simulink model "GesamtsystemAlt"  (R2018b)
settings: Solver=FixedStepDiscrete  StartTime=0.0  StopTime=1  RelTol=1e-3  EnableMultiTasking=on
libraries: commutil2 x12, c2833xlib x10, c280xlib x8, powerlib_extras x2, simulink x1, c2000lib x1, dspstat3 x1
(part 1 of 3)
settings Model: ExtModeTrigDuration=8  Creator=User  LastModifiedBy=User
settings SolverCC: AutoInsertRateTranBlk=on
settings DataIOCC: LimitDataPoints=on  SaveFormat=Array  SaveOutput=off  SaveTime=off
settings OptimizationCC: DefaultUnderspecifiedDataType=single  ExpressionDepthLimit=2147483647  LifeSpan=1  MaxStackSize=512
settings DebuggingCC: UnderspecifiedInitializationDetection=Classic  MergeDetectMultiDrivingBlocksExec=none  SolverPrmCheckMsg=warning  StateNameClashWarn=warning  SFUnexpectedBacktrackingDiag=warning  SFNoUnconditionalDefaultTransitionDiag=warning  SFExecutionAtInitializationDiag=none
settings HardwareCC: ProdBitPerChar=16  ProdBitPerInt=16  ProdBitPerPointer=32  ProdBitPerSizeT=32  ProdBitPerPtrDiffT=32  ProdLargestAtomicInteger=Integer  ProdLargestAtomicFloat=None  ProdWordSize=16  ProdLongLongMode=on  ProdHWDeviceType=Texas Instruments->C2000  TargetBitPerChar=16  TargetBitPerInt=16  TargetLargestAtomicInteger=Integer  TargetIntDivRoundTo=Zero  TargetEndianess=LittleEndian  TargetWordSize=16  TargetHWDeviceType=Texas Instruments->C2000  ProdEqTarget=off
settings ModelReferenceCC: PropagateSignalLabelsOutOfModel=off
settings SFSimCC: SimCustomSourceCode="#include \"i2c_reset.c\""  SimCustomHeaderCode="#include \"i2c_reset.h\""  SimUseLocalCustomCode=off  MATLABDynamicMemAlloc=off
settings RTWCC: SystemTargetFile=ert.tlc  HardwareBoard=TI Delfino F2833x  TemplateMakefile=ert_default_tmf  RTWUseLocalCustomCode=off  RTWUseSimCustomCode=on  CustomSourceCode="#include \"i2c_reset.c\""  CustomHeaderCode="#include \"i2c_reset.h\""  Toolchain=Texas Instruments Code Composer Studio (C2000)
settings CodeAppCC: IgnoreCustomStorageClasses=off  CustomSymbolStrType=$N$R$M  StateflowObjectComments=on  InternalIdentifier=Classic
settings ERTTargetCC: CodeReplacementLibrary=TI C28x  MultiwordLength=2048  ParMdlRefBuildCompliant=off  SupportContinuousTime=on  CPPClassGenCompliant=off  ConvertIfToSwitch=off  SuppressUnreachableDefaultCases=off
settings ConfigComp: CovMetricSettings=dw  CovHtmlReporting=on  CovSaveCumulativeToWorkspaceVar=on  CovSaveSingleToWorkspaceVar=on  CovExternalEMLEnable=off  PSAutoStubLUT=on

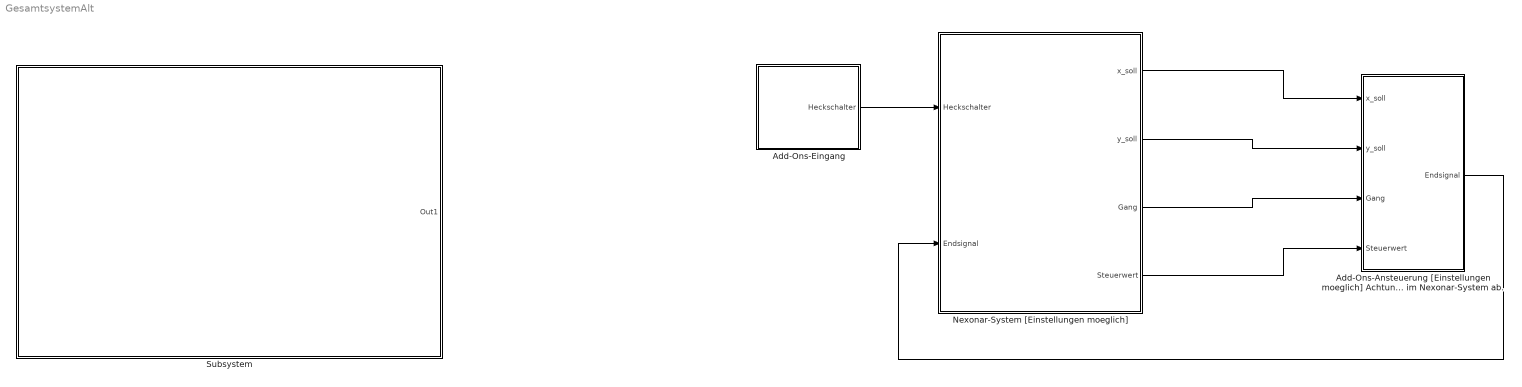
== system GesamtsystemAlt ==
  Add-Ons-Ansteuerung [Einstellungen moeglich] Achtung! Einige Einstellungswerte haengen von den Werten im Nexonar-System ab. : Subsystem
  Add-Ons-Eingang : Subsystem
  Nexonar-System [Einstellungen moeglich] : Subsystem
  Subsystem : Subsystem
  wires:
  Add-Ons-Eingang/1(Heckschalter) -> Nexonar-System [Einstellungen moeglich]/1(Heckschalter)
  Nexonar-System [Einstellungen moeglich]/1(x_soll) -> Add-Ons-Ansteuerung [Einstellungen moeglich] Achtung! Einige Einstellungswerte haengen von den Werten im Nexonar-System ab./1(x_soll)
  Nexonar-System [Einstellungen moeglich]/4(Steuerwert) -> Add-Ons-Ansteuerung [Einstellungen moeglich] Achtung! Einige Einstellungswerte haengen von den Werten im Nexonar-System ab./4(Steuerwert)
  Nexonar-System [Einstellungen moeglich]/3(Gang) -> Add-Ons-Ansteuerung [Einstellungen moeglich] Achtung! Einige Einstellungswerte haengen von den Werten im Nexonar-System ab./3(Gang)
  Nexonar-System [Einstellungen moeglich]/2(y_soll) -> Add-Ons-Ansteuerung [Einstellungen moeglich] Achtung! Einige Einstellungswerte haengen von den Werten im Nexonar-System ab./2(y_soll)
  Add-Ons-Ansteuerung [Einstellungen moeglich] Achtung! Einige Einstellungswerte haengen von den Werten im Nexonar-System ab./1(Endsignal) -> Nexonar-System [Einstellungen moeglich]/2(Endsignal)

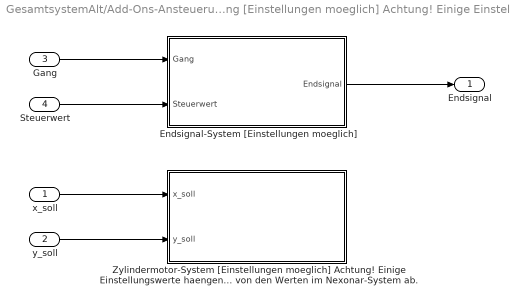
== system GesamtsystemAlt/Add-Ons-Ansteuerung [Einstellungen moeglich] Achtung! Einige Einstellungswerte haengen von den Werten im Nexonar-System ab. ==
  x_soll : Inport
  y_soll : Inport  Port=2
  Gang : Inport  Port=3
  Steuerwert : Inport  Port=4
  Endsignal-System [Einstellungen moeglich] : Subsystem
  Zylindermotor-System [Einstellungen moeglich] Achtung! Einige Einstellungswerte haengen von den Werten im Nexonar-System ab. : Subsystem
  Endsignal : Outport
  wires:
  x_soll/1 -> Zylindermotor-System [Einstellungen moeglich] Achtung! Einige Einstellungswerte haengen von den Werten im Nexonar-System ab./1(x_soll)
  y_soll/1 -> Zylindermotor-System [Einstellungen moeglich] Achtung! Einige Einstellungswerte haengen von den Werten im Nexonar-System ab./2(y_soll)
  Gang/1 -> Endsignal-System [Einstellungen moeglich]/1(Gang)
  Steuerwert/1 -> Endsignal-System [Einstellungen moeglich]/2(Steuerwert)
  Endsignal-System [Einstellungen moeglich]/1(Endsignal) -> Endsignal/1

== system GesamtsystemAlt/Add-Ons-Eingang ==
  Heckschalter-System : Subsystem
  Heckschalter : Outport
  wires:
  Heckschalter-System/1(Heckschalter) -> Heckschalter/1

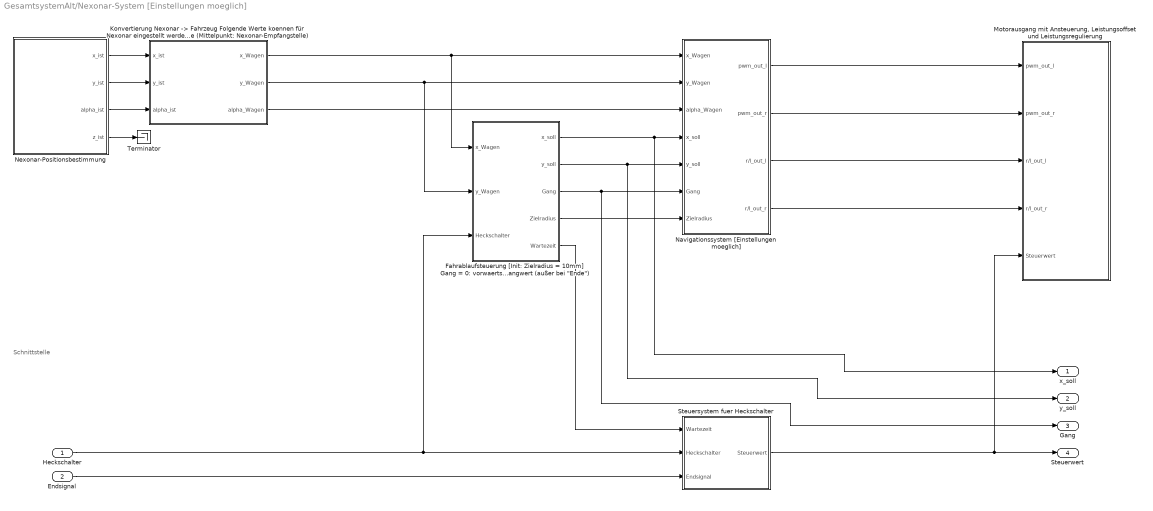
== system GesamtsystemAlt/Nexonar-System [Einstellungen moeglich] ==
  note: Schnittstelle
  Heckschalter : Inport
  Endsignal : Inport  Port=2
  "Fahrablaufsteuerung [Init: Zielradius = 10mm] Gang = 0: vorwaerts Gang = 1: rueckwaerts Folgende Werte fuer den Ablauf sind einstellbar: - Zielkoordinatenwerte - Gangwert (außer bei \"Ende\")" : Stateflow chart  TreatAsAtomicUnit=on
  "Konvertierung Nexonar -> Fahrzeug Folgende Werte koennen für Nexonar eingestellt werden: - r_Versatz_Nexo: Radialer Versatz des Nexonars zur Rotationsachse des Fahrzeugs - phi_Versatz_Nexo: Winkelversatz des Nexonars gegenüber der x-Achse (Mittelpunkt: Rotationspunkt des Fahrzeugs) - psi_Offset_Nexo: Winkelversatz des Nexonars gegenüber der x-Achse (Mittelpunkt: Nexonar-Empfangstelle)" : Stateflow chart  TreatAsAtomicUnit=on
  "Motorausgang mit Ansteuerung, Leistungsoffset und Leistungsregulierung" : Subsystem
  Navigationssystem [Einstellungen moeglich] : Subsystem  TreatAsAtomicUnit=on
  Nexonar-Positionsbestimmung : Subsystem
  Steuersystem fuer Heckschalter : Stateflow chart  TreatAsAtomicUnit=on
  Terminator : Terminator
  x_soll : Outport
  y_soll : Outport  Port=2
  Gang : Outport  Port=3
  Steuerwert : Outport  Port=4
  wires:
  Navigationssystem [Einstellungen moeglich]/3(r/l_out_l) -> "Motorausgang mit Ansteuerung, Leistungsoffset und Leistungsregulierung"/3(r/l_out_l)
  "Konvertierung Nexonar -> Fahrzeug Folgende Werte koennen für Nexonar eingestellt werden: - r_Versatz_Nexo: Radialer Versatz des Nexonars zur Rotationsachse des Fahrzeugs - phi_Versatz_Nexo: Winkelversatz des Nexonars gegenüber der x-Achse (Mittelpunkt: Rotationspunkt des Fahrzeugs) - psi_Offset_Nexo: Winkelversatz des Nexonars gegenüber der x-Achse (Mittelpunkt: Nexonar-Empfangstelle)"/2(y_Wagen) -> "Fahrablaufsteuerung [Init: Zielradius = 10mm] Gang = 0: vorwaerts Gang = 1: rueckwaerts Folgende Werte fuer den Ablauf sind einstellbar: - Zielkoordinatenwerte - Gangwert (außer bei \"Ende\")"/2(y_Wagen), Navigationssystem [Einstellungen moeglich]/2(y_Wagen)
  "Konvertierung Nexonar -> Fahrzeug Folgende Werte koennen für Nexonar eingestellt werden: - r_Versatz_Nexo: Radialer Versatz des Nexonars zur Rotationsachse des Fahrzeugs - phi_Versatz_Nexo: Winkelversatz des Nexonars gegenüber der x-Achse (Mittelpunkt: Rotationspunkt des Fahrzeugs) - psi_Offset_Nexo: Winkelversatz des Nexonars gegenüber der x-Achse (Mittelpunkt: Nexonar-Empfangstelle)"/1(x_Wagen) -> "Fahrablaufsteuerung [Init: Zielradius = 10mm] Gang = 0: vorwaerts Gang = 1: rueckwaerts Folgende Werte fuer den Ablauf sind einstellbar: - Zielkoordinatenwerte - Gangwert (außer bei \"Ende\")"/1(x_Wagen), Navigationssystem [Einstellungen moeglich]/1(x_Wagen)
  Nexonar-Positionsbestimmung/4(z_ist) -> Terminator/1
  Nexonar-Positionsbestimmung/1(x_ist) -> "Konvertierung Nexonar -> Fahrzeug Folgende Werte koennen für Nexonar eingestellt werden: - r_Versatz_Nexo: Radialer Versatz des Nexonars zur Rotationsachse des Fahrzeugs - phi_Versatz_Nexo: Winkelversatz des Nexonars gegenüber der x-Achse (Mittelpunkt: Rotationspunkt des Fahrzeugs) - psi_Offset_Nexo: Winkelversatz des Nexonars gegenüber der x-Achse (Mittelpunkt: Nexonar-Empfangstelle)"/1(x_ist)
  Navigationssystem [Einstellungen moeglich]/4(r/l_out_r) -> "Motorausgang mit Ansteuerung, Leistungsoffset und Leistungsregulierung"/4(r/l_out_r)
  Nexonar-Positionsbestimmung/3(alpha_ist) -> "Konvertierung Nexonar -> Fahrzeug Folgende Werte koennen für Nexonar eingestellt werden: - r_Versatz_Nexo: Radialer Versatz des Nexonars zur Rotationsachse des Fahrzeugs - phi_Versatz_Nexo: Winkelversatz des Nexonars gegenüber der x-Achse (Mittelpunkt: Rotationspunkt des Fahrzeugs) - psi_Offset_Nexo: Winkelversatz des Nexonars gegenüber der x-Achse (Mittelpunkt: Nexonar-Empfangstelle)"/3(alpha_ist)
  "Konvertierung Nexonar -> Fahrzeug Folgende Werte koennen für Nexonar eingestellt werden: - r_Versatz_Nexo: Radialer Versatz des Nexonars zur Rotationsachse des Fahrzeugs - phi_Versatz_Nexo: Winkelversatz des Nexonars gegenüber der x-Achse (Mittelpunkt: Rotationspunkt des Fahrzeugs) - psi_Offset_Nexo: Winkelversatz des Nexonars gegenüber der x-Achse (Mittelpunkt: Nexonar-Empfangstelle)"/3(alpha_Wagen) -> Navigationssystem [Einstellungen moeglich]/3(alpha_Wagen)
  "Fahrablaufsteuerung [Init: Zielradius = 10mm] Gang = 0: vorwaerts Gang = 1: rueckwaerts Folgende Werte fuer den Ablauf sind einstellbar: - Zielkoordinatenwerte - Gangwert (außer bei \"Ende\")"/4(Zielradius) -> Navigationssystem [Einstellungen moeglich]/7(Zielradius)
  Nexonar-Positionsbestimmung/2(y_ist) -> "Konvertierung Nexonar -> Fahrzeug Folgende Werte koennen für Nexonar eingestellt werden: - r_Versatz_Nexo: Radialer Versatz des Nexonars zur Rotationsachse des Fahrzeugs - phi_Versatz_Nexo: Winkelversatz des Nexonars gegenüber der x-Achse (Mittelpunkt: Rotationspunkt des Fahrzeugs) - psi_Offset_Nexo: Winkelversatz des Nexonars gegenüber der x-Achse (Mittelpunkt: Nexonar-Empfangstelle)"/2(y_ist)
  Navigationssystem [Einstellungen moeglich]/1(pwm_out_l) -> "Motorausgang mit Ansteuerung, Leistungsoffset und Leistungsregulierung"/1(pwm_out_l)
  Navigationssystem [Einstellungen moeglich]/2(pwm_out_r) -> "Motorausgang mit Ansteuerung, Leistungsoffset und Leistungsregulierung"/2(pwm_out_r)
  "Fahrablaufsteuerung [Init: Zielradius = 10mm] Gang = 0: vorwaerts Gang = 1: rueckwaerts Folgende Werte fuer den Ablauf sind einstellbar: - Zielkoordinatenwerte - Gangwert (außer bei \"Ende\")"/5(Wartezeit) -> Steuersystem fuer Heckschalter/1(Wartezeit)
  Steuersystem fuer Heckschalter/1(Steuerwert) -> Steuerwert/1, "Motorausgang mit Ansteuerung, Leistungsoffset und Leistungsregulierung"/5(Steuerwert)
  Heckschalter/1 -> Steuersystem fuer Heckschalter/2(Heckschalter), "Fahrablaufsteuerung [Init: Zielradius = 10mm] Gang = 0: vorwaerts Gang = 1: rueckwaerts Folgende Werte fuer den Ablauf sind einstellbar: - Zielkoordinatenwerte - Gangwert (außer bei \"Ende\")"/3(Heckschalter)
  "Fahrablaufsteuerung [Init: Zielradius = 10mm] Gang = 0: vorwaerts Gang = 1: rueckwaerts Folgende Werte fuer den Ablauf sind einstellbar: - Zielkoordinatenwerte - Gangwert (außer bei \"Ende\")"/2(y_soll) -> y_soll/1, Navigationssystem [Einstellungen moeglich]/5(y_soll)
  "Fahrablaufsteuerung [Init: Zielradius = 10mm] Gang = 0: vorwaerts Gang = 1: rueckwaerts Folgende Werte fuer den Ablauf sind einstellbar: - Zielkoordinatenwerte - Gangwert (außer bei \"Ende\")"/3(Gang) -> Gang/1, Navigationssystem [Einstellungen moeglich]/6(Gang)
  "Fahrablaufsteuerung [Init: Zielradius = 10mm] Gang = 0: vorwaerts Gang = 1: rueckwaerts Folgende Werte fuer den Ablauf sind einstellbar: - Zielkoordinatenwerte - Gangwert (außer bei \"Ende\")"/1(x_soll) -> x_soll/1, Navigationssystem [Einstellungen moeglich]/4(x_soll)
  Endsignal/1 -> Steuersystem fuer Heckschalter/3(Endsignal)

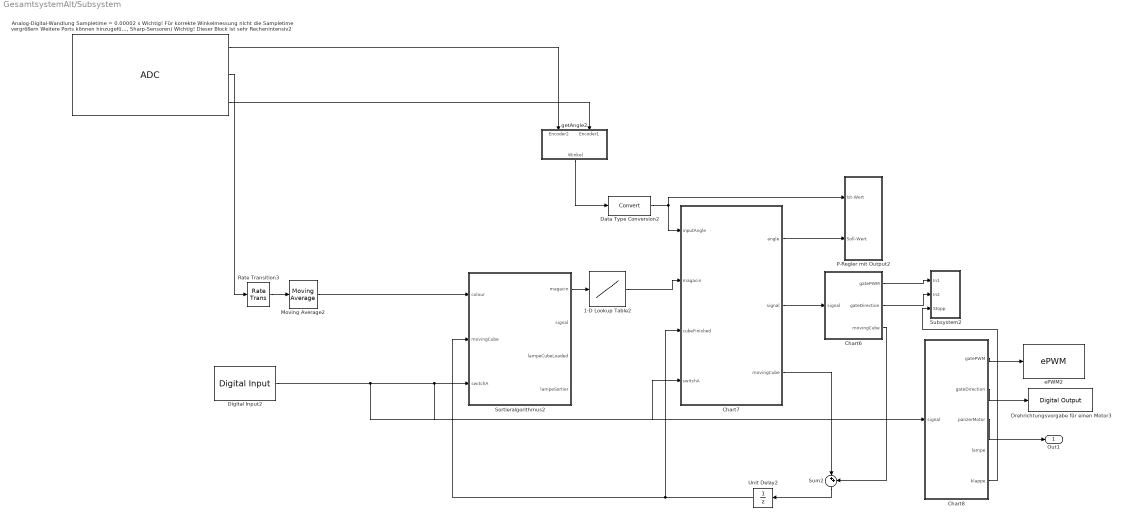
== system GesamtsystemAlt/Subsystem ==
  1-D Lookup Table2 : Lookup_n-D  NumberOfTableDimensions=1  BreakpointsForDimension1=[-1,0,1,2,3,4,5,6]  Table=[-1,-440,-295,-170,-40,85,220,430]  InternalRulePriority=Speed  RndMeth=Simplest  InputSameDT=on
  "Analog-Digital-Wandlung Sampletime = 0.00002 s Wichtig! Für korrekte Winkelmessung nicht die Sampletime vergrößern Weitere Ports können hinzugefügt werden (Farbsensor, Sharp-Sensoren) Wichtig! Dieser Block ist sehr Rechenintensiv2" : c280xlib/ADC  useModule=A  useMode=Sequential  sourceSOC=Software  sourceSOC1=Software  sourceSOC2=ePWMxB  xint2_ADCSOC=31  Ts=0.00002  dType=double  postInterrupt=off  numConversionsSingle=3  numConversionsDouble=1  conv0=ADCINA0  conv1=ADCINA1  conv2=ADCINA2  conv3=ADCINA3  conv4=ADCINA4  conv5=ADCINA5  conv6=ADCINA6  conv7=ADCINA7  conv8=ADCINB0  conv9=ADCINB1  conv10=ADCINB2  conv11=ADCINB3  conv12=ADCINB4  conv13=ADCINB5  conv14=ADCINB6  conv15=ADCINB7  convAB0=ADCINA0 and ADCINB0  convAB1=ADCINA1 and ADCINB1  convAB2=ADCINA2 and ADCINB2  convAB3=ADCINA3 and ADCINB3  convAB4=ADCINA4 and ADCINB4  convAB5=ADCINA5 and ADCINB5  convAB6=ADCINA6 and ADCINB6  convAB7=ADCINA7 and ADCINB7  convA0=ADCINA1  convA1=ADCINA2  convA2=ADCINA0  convA3=ADCINA1  convA4=ADCINA5  convA5=ADCINA5  convA6=ADCINA6  convA7=ADCINA7  convB0=ADCINB0  convB1=ADCINB1  convB2=ADCINB2  convB3=ADCINB3  convB4=ADCINB4  convB5=ADCINB5  convB6=ADCINB6  convB7=ADCINB7  c28xmultiPort=on  endma=off  chdma=1
      settings: SourceProductName=Embedded Coder Support Package for Texas Instruments C2000 Processors  SourceProductBaseCode=TIC2000
  Chart6 : Stateflow chart  TreatAsAtomicUnit=on
  Chart7 : Stateflow chart  TreatAsAtomicUnit=on
  Chart8 : Stateflow chart  TreatAsAtomicUnit=on
  Data Type Conversion2 : DataTypeConversion
  Digital Input2 : c2833xlib/Digital Input  GPIO_Number=GPIO24~GPIO31  GPIO_Bit0=on  GPIO_Bit1=off  GPIO_Bit2=off  GPIO_Bit3=off  GPIO_Bit4=off  GPIO_Bit5=off  GPIO_Bit6=off  GPIO_Bit7=off  sampleTime=0.1  dataType=auto  GPIO_Bit0_Qualification=Sync to SYSCLKOUT  GPIO_Bit1_Qualification=Sync to SYSCLKOUT  GPIO_Bit2_Qualification=Sync to SYSCLKOUT  GPIO_Bit3_Qualification=Sync to SYSCLKOUT  GPIO_Bit4_Qualification=Sync to SYSCLKOUT  GPIO_Bit5_Qualification=Sync to SYSCLKOUT  GPIO_Bit6_Qualification=Sync to SYSCLKOUT  GPIO_Bit7_Qualification=Sync to SYSCLKOUT  Qualification_Period=-1
      settings: SourceProductName=Embedded Coder Support Package for Texas Instruments C2000 Processors  SourceProductBaseCode=TIC2000
  Drehrichtungsvorgabe für einen Motor3 : c2833xlib/Digital Output  GPIO_Number=GPIO8~GPIO15  GPIO_Bit0=off  GPIO_BIT0_Toggle=off  GPIO_Bit1=off  GPIO_BIT1_Toggle=off  GPIO_Bit2=off  GPIO_BIT2_Toggle=off  GPIO_Bit3=off  GPIO_BIT3_Toggle=off  GPIO_Bit4=off  GPIO_BIT4_Toggle=off  GPIO_Bit5=off  GPIO_BIT5_Toggle=off  GPIO_Bit6=off  GPIO_BIT6_Toggle=off  GPIO_Bit7=on  GPIO_BIT7_Toggle=off
      settings: SourceProductName=Embedded Coder Support Package for Texas Instruments C2000 Processors  SourceProductBaseCode=TIC2000
  Moving Average2 : dspstat3/Moving Average  Method=Exponential weighting  ForgettingFactorPort=off  SpecifyWindowLength=on  WindowLength=4  ForgettingFactor=0.3  SimulateUsing=Code generation
  P-Regler mit Output2 : Subsystem
  Rate Transition3 : RateTransition  OutPortSampleTime=0.01
  Sortieralgorithmus2 : Stateflow chart  TreatAsAtomicUnit=on
  Subsystem2 : Subsystem
  Sum2 : Sum  Inputs=|++
  Unit Delay2 : UnitDelay  SampleTime=-1
  ePWM2 : c280xlib/ePWM  checkMode=off  useModule=ePWM5  periodUnits=Clock cycles  timerSource=Specify via dialog  timerPeriod_clk=64000  timerPeriod_sec=0.0001  tbshadow=Counter equals to zero  countingMode=Up  phaseActiveEnable=Disable  phaseDirection=Count down after sync  phaseActive=0  synchronizationEnable=off  synchronizationOption=Disable  clockPrescale=1  HSclockPrescale=1  ePWMxAStatus=off  CMPAUnits=Clock cycles  CMPASource=Specify via dialog  CMPAValue_per=50  CMPAValue_clk=32000  enCMPAshadow=Counter equals to zero  ePWMxAactionLogic1=Do nothing  ePWMxAactionLogic2=Clear  ePWMxAactionLogic3=Set  ePWMxAactionLogic4=Do nothing  ePWMxAactionLogic5=Do nothing  ePWMxAactionLogic6=Do nothing  ePWMxALoadMode=Load on counter equals to zero (CTR=Zero)  ePWMxACSFenable=off  ePWMxACSFvalue=Forcing disable  ePWMxASFreload=Zero  enHRPWM=off  HRPWM_LoadMode=Counter equals to zero (CTR=ZERO)  HRPWM_CTLMode=Phase control mode  HRPWM_EDGMode=Both edge  enSFO=on  ePWMxBStatus=on  CMPBUnits=Percentages  CMPBSource=Input port  CMPBValue_per=50  CMPBValue_clk=32000  enCMPBshadow=Counter equals to zero  ePWMxBactionLogic1=Do nothing  ePWMxBactionLogic2=Set  ePWMxBactionLogic3=Do nothing  ePWMxBactionLogic4=Do nothing  ePWMxBactionLogic5=Clear  ePWMxBactionLogic6=Do nothing  ePWMxBLoadMode=Load on counter equals to zero (CTR=Zero)  ePWMxBCSFenable=off  ePWMxBCSFvalue=Forcing disable  ePWMxBSFreload=Zero  enableDBePWMxA=off  enableDBePWMxB=off  DBpolarity=Active high (AH)  DBedgeDelay=Positive  DBSource_ePWMxA=ePWMxA  DBSource_ePWMxB=ePWMxA  DBperiodSource=Specify via dialog  REDperiod=0  FEDperiod=0  adcstartModuleA=off  adcrequestEventA=First event  adcstartEventA=Counter equals to zero (CTR=Zero)  adcstartModuleB=off  adcrequestEventB=First event  adcstartEventB=Counter equals to zero (CTR=Zero)  intEn=off  intPrd=First event  intSel=Counter equals to zero (CTR=Zero)  chopperEnable=off  chopperFrequency=1  chopperFirstwidth=1  chopperDuty=12.5%  tripZonesource=Specify via dialog  tzselOSHT1=off  tzselOSHT2=off  tzselOSHT3=off  tzselOSHT4=off  tzselOSHT5=off  tzselOSHT6=off  tzselCBC1=off  tzselCBC2=off  tzselCBC3=off  tzselCBC4=off  tzselCBC5=off  tzselCBC6=off  enTzOstIntr=off  enTzCbcIntr=off  ePWMxAforced=No action  ePWMxBforced=No action  timerPeriod=-1  ePWMxAValue=0  ePWMxBValue=0  tripZoneoption=One-shot trip (OSHT)
      settings: SourceProductName=Embedded Coder Support Package for Texas Instruments C2000 Processors  SourceProductBaseCode=TIC2000
  getAngle2 : Subsystem
  Out1 : Outport
  wires:
  Moving Average2/1 -> Sortieralgorithmus2/1(colour)
  Chart8/1(gatePWM) -> ePWM2/1
  getAngle2/1(Winkel) -> Data Type Conversion2/1
  Chart6/3(movingCube) -> Sum2/2
  "Analog-Digital-Wandlung Sampletime = 0.00002 s Wichtig! Für korrekte Winkelmessung nicht die Sampletime vergrößern Weitere Ports können hinzugefügt werden (Farbsensor, Sharp-Sensoren) Wichtig! Dieser Block ist sehr Rechenintensiv2"/2 -> Rate Transition3/1
  Digital Input2/1 -> Chart7/4(switchA), Chart8/1(signal), Sortieralgorithmus2/3(switchA)
  Chart6/1(gatePWM) -> Subsystem2/1(In1)
  Chart8/2(gateDirection) -> Drehrichtungsvorgabe für einen Motor3/1
  Chart7/1(angle) -> P-Regler mit Output2/2(Soll-Wert)
  Rate Transition3/1 -> Moving Average2/1
  Unit Delay2/1 -> Chart7/3(cubeFinished), Sortieralgorithmus2/2(movingCube)
  Chart6/2(gateDirection) -> Subsystem2/2(In2)
  Data Type Conversion2/1 -> Chart7/1(inputAngle), P-Regler mit Output2/1(Ist-Wert)
  Sortieralgorithmus2/1(magacin) -> 1-D Lookup Table2/1
  Chart7/2(signal) -> Chart6/1(signal)
  1-D Lookup Table2/1 -> Chart7/2(magacin)
  "Analog-Digital-Wandlung Sampletime = 0.00002 s Wichtig! Für korrekte Winkelmessung nicht die Sampletime vergrößern Weitere Ports können hinzugefügt werden (Farbsensor, Sharp-Sensoren) Wichtig! Dieser Block ist sehr Rechenintensiv2"/1 -> getAngle2/1(Encoder2)
  Sum2/1 -> Unit Delay2/1
  Chart7/3(movingCube) -> Sum2/1
  "Analog-Digital-Wandlung Sampletime = 0.00002 s Wichtig! Für korrekte Winkelmessung nicht die Sampletime vergrößern Weitere Ports können hinzugefügt werden (Farbsensor, Sharp-Sensoren) Wichtig! Dieser Block ist sehr Rechenintensiv2"/3 -> getAngle2/2(Encoder1)
  Chart8/3(panzerMotor) -> Out1/1
  Chart8/5(klappe) -> Subsystem2/3("Stopp ")

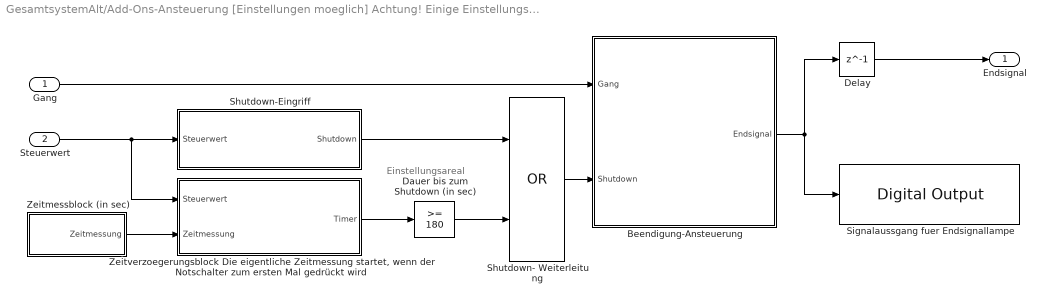
== system GesamtsystemAlt/Add-Ons-Ansteuerung [Einstellungen moeglich] Achtung! Einige Einstellungswerte haengen von den Werten im Nexonar-System ab./Endsignal-System [Einstellungen moeglich] ==
  note: Einstellungsareal
  Gang : Inport
  Steuerwert : Inport  Port=2
  Beendigung-Ansteuerung : Stateflow chart  TreatAsAtomicUnit=on
  Dauer bis zum Shutdown (in sec) : simulink/Logic and Bit Operations/Compare To Constant  relop=>=  const=180  OutDataTypeStr=boolean
  Delay : Delay  DelayLength=1  InitialCondition=0
  Shutdown- Weiterleitung : Logic  Operator=OR  AllPortsSameDT=off  OutDataTypeStr=boolean
  Shutdown-Eingriff : Stateflow chart  TreatAsAtomicUnit=on
  Signalaussgang fuer Endsignallampe : c2833xlib/Digital Output  GPIO_Number=GPIO56~GPIO63  GPIO_Bit0=off  GPIO_BIT0_Toggle=off  GPIO_Bit1=off  GPIO_BIT1_Toggle=off  GPIO_Bit2=on  GPIO_BIT2_Toggle=off  GPIO_Bit3=off  GPIO_BIT3_Toggle=off  GPIO_Bit4=off  GPIO_BIT4_Toggle=off  GPIO_Bit5=off  GPIO_BIT5_Toggle=off  GPIO_Bit6=off  GPIO_BIT6_Toggle=off  GPIO_Bit7=off  GPIO_BIT7_Toggle=off
      settings: SourceProductName=Embedded Coder Support Package for Texas Instruments C2000 Processors  SourceProductBaseCode=TIC2000
  Zeitmessblock (in sec) : Subsystem
  "Zeitverzoegerungsblock Die eigentliche Zeitmessung startet, wenn der Notschalter zum ersten Mal gedrückt wird" : Stateflow chart  TreatAsAtomicUnit=on
  Endsignal : Outport
  wires:
  Gang/1 -> Beendigung-Ansteuerung/1(Gang)
  Beendigung-Ansteuerung/1(Endsignal) -> Signalaussgang fuer Endsignallampe/1, Delay/1
  "Zeitverzoegerungsblock Die eigentliche Zeitmessung startet, wenn der Notschalter zum ersten Mal gedrückt wird"/1(Timer) -> Dauer bis zum Shutdown (in sec)/1
  Steuerwert/1 -> "Zeitverzoegerungsblock Die eigentliche Zeitmessung startet, wenn der Notschalter zum ersten Mal gedrückt wird"/1(Steuerwert), Shutdown-Eingriff/1(Steuerwert)
  Zeitmessblock (in sec)/1(Zeitmessung) -> "Zeitverzoegerungsblock Die eigentliche Zeitmessung startet, wenn der Notschalter zum ersten Mal gedrückt wird"/2(Zeitmessung)
  Delay/1 -> Endsignal/1
  Shutdown- Weiterleitung/1 -> Beendigung-Ansteuerung/2(Shutdown)
  Dauer bis zum Shutdown (in sec)/1 -> Shutdown- Weiterleitung/2
  Shutdown-Eingriff/1(Shutdown) -> Shutdown- Weiterleitung/1

== system GesamtsystemAlt/Add-Ons-Ansteuerung [Einstellungen moeglich] Achtung! Einige Einstellungswerte haengen von den Werten im Nexonar-System ab./Zylindermotor-System [Einstellungen moeglich] Achtung! Einige Einstellungswerte haengen von den Werten im Nexonar-System ab. ==
  x_soll : Inport
  y_soll : Inport  Port=2
  Drehrichtungsvorgabe für Zylindermotor : c2833xlib/Digital Output  GPIO_Number=GPIO16~GPIO23  GPIO_Bit0=off  GPIO_BIT0_Toggle=off  GPIO_Bit1=on  GPIO_BIT1_Toggle=off  GPIO_Bit2=off  GPIO_BIT2_Toggle=off  GPIO_Bit3=off  GPIO_BIT3_Toggle=off  GPIO_Bit4=off  GPIO_BIT4_Toggle=off  GPIO_Bit5=off  GPIO_BIT5_Toggle=off  GPIO_Bit6=off  GPIO_BIT6_Toggle=off  GPIO_Bit7=off  GPIO_BIT7_Toggle=off
      settings: SourceProductName=Embedded Coder Support Package for Texas Instruments C2000 Processors  SourceProductBaseCode=TIC2000
  PWM Vorgabe für Zylindermotor : c280xlib/ePWM  checkMode=off  useModule=ePWM3  periodUnits=Clock cycles  timerSource=Specify via dialog  timerPeriod_clk=64000  timerPeriod_sec=0.0001  tbshadow=Counter equals to zero  countingMode=Up  phaseActiveEnable=Disable  phaseDirection=Count down after sync  phaseActive=0  synchronizationEnable=off  synchronizationOption=Disable  clockPrescale=1  HSclockPrescale=1  ePWMxAStatus=off  CMPAUnits=Clock cycles  CMPASource=Specify via dialog  CMPAValue_per=50  CMPAValue_clk=32000  enCMPAshadow=Counter equals to zero  ePWMxAactionLogic1=Do nothing  ePWMxAactionLogic2=Clear  ePWMxAactionLogic3=Set  ePWMxAactionLogic4=Do nothing  ePWMxAactionLogic5=Do nothing  ePWMxAactionLogic6=Do nothing  ePWMxALoadMode=Load on counter equals to zero (CTR=Zero)  ePWMxACSFenable=off  ePWMxACSFvalue=Forcing disable  ePWMxASFreload=Zero  enHRPWM=off  HRPWM_LoadMode=Counter equals to zero (CTR=ZERO)  HRPWM_CTLMode=Phase control mode  HRPWM_EDGMode=Both edge  enSFO=on  ePWMxBStatus=on  CMPBUnits=Percentages  CMPBSource=Input port  CMPBValue_per=0  CMPBValue_clk=32000  enCMPBshadow=Counter equals to zero  ePWMxBactionLogic1=Do nothing  ePWMxBactionLogic2=Set  ePWMxBactionLogic3=Do nothing  ePWMxBactionLogic4=Do nothing  ePWMxBactionLogic5=Clear  ePWMxBactionLogic6=Do nothing  ePWMxBLoadMode=Load on counter equals to zero (CTR=Zero)  ePWMxBCSFenable=off  ePWMxBCSFvalue=Forcing disable  ePWMxBSFreload=Zero  enableDBePWMxA=off  enableDBePWMxB=off  DBpolarity=Active high (AH)  DBedgeDelay=Positive  DBSource_ePWMxA=ePWMxA  DBSource_ePWMxB=ePWMxA  DBperiodSource=Specify via dialog  REDperiod=0  FEDperiod=0  adcstartModuleA=off  adcrequestEventA=First event  adcstartEventA=Counter equals to zero (CTR=Zero)  adcstartModuleB=off  adcrequestEventB=First event  adcstartEventB=Counter equals to zero (CTR=Zero)  intEn=off  intPrd=First event  intSel=Counter equals to zero (CTR=Zero)  chopperEnable=off  chopperFrequency=1  chopperFirstwidth=1  chopperDuty=12.5%  tripZonesource=Specify via dialog  tzselOSHT1=off  tzselOSHT2=off  tzselOSHT3=off  tzselOSHT4=off  tzselOSHT5=off  tzselOSHT6=off  tzselCBC1=off  tzselCBC2=off  tzselCBC3=off  tzselCBC4=off  tzselCBC5=off  tzselCBC6=off  enTzOstIntr=off  enTzCbcIntr=off  ePWMxAforced=No action  ePWMxBforced=No action  timerPeriod=-1  ePWMxAValue=0  ePWMxBValue=0  tripZoneoption=One-shot trip (OSHT)
      settings: SourceProductName=Embedded Coder Support Package for Texas Instruments C2000 Processors  SourceProductBaseCode=TIC2000
  "Zylindermotor-Ansteuerung Folgende Werte sind einstellbar: - Drehstaerke (in %) (-> ZM_pwm_out in \"Ausfuerung\") - Drehrichtung (rechts = 0, links = 1) (-> ZM_r_l_out in \"Init_und_Warten\") - Drehdauer (-> zwischen \"Ausfuehrung\" und \"Beendet\") - Ausfuehrungspunkt (in mm) [durch Wechsel der Soll-Position] (-> zwischen \"Init_und_Start\" und \"Ausfuehrung) Wichtig! Der Ausfuerungspunkt haengt von den EXAKTEN Soll-Werten aus der Fahrablaufsteuerung im Nexonar-System ab." : Stateflow chart  TreatAsAtomicUnit=on
  wires:
  "Zylindermotor-Ansteuerung Folgende Werte sind einstellbar: - Drehstaerke (in %) (-> ZM_pwm_out in \"Ausfuerung\") - Drehrichtung (rechts = 0, links = 1) (-> ZM_r_l_out in \"Init_und_Warten\") - Drehdauer (-> zwischen \"Ausfuehrung\" und \"Beendet\") - Ausfuehrungspunkt (in mm) [durch Wechsel der Soll-Position] (-> zwischen \"Init_und_Start\" und \"Ausfuehrung) Wichtig! Der Ausfuerungspunkt haengt von den EXAKTEN Soll-Werten aus der Fahrablaufsteuerung im Nexonar-System ab."/1(ZM_pwm_out) -> PWM Vorgabe für Zylindermotor/1
  "Zylindermotor-Ansteuerung Folgende Werte sind einstellbar: - Drehstaerke (in %) (-> ZM_pwm_out in \"Ausfuerung\") - Drehrichtung (rechts = 0, links = 1) (-> ZM_r_l_out in \"Init_und_Warten\") - Drehdauer (-> zwischen \"Ausfuehrung\" und \"Beendet\") - Ausfuehrungspunkt (in mm) [durch Wechsel der Soll-Position] (-> zwischen \"Init_und_Start\" und \"Ausfuehrung) Wichtig! Der Ausfuerungspunkt haengt von den EXAKTEN Soll-Werten aus der Fahrablaufsteuerung im Nexonar-System ab."/2(ZM_r_l_out) -> Drehrichtungsvorgabe für Zylindermotor/1
  y_soll/1 -> "Zylindermotor-Ansteuerung Folgende Werte sind einstellbar: - Drehstaerke (in %) (-> ZM_pwm_out in \"Ausfuerung\") - Drehrichtung (rechts = 0, links = 1) (-> ZM_r_l_out in \"Init_und_Warten\") - Drehdauer (-> zwischen \"Ausfuehrung\" und \"Beendet\") - Ausfuehrungspunkt (in mm) [durch Wechsel der Soll-Position] (-> zwischen \"Init_und_Start\" und \"Ausfuehrung) Wichtig! Der Ausfuerungspunkt haengt von den EXAKTEN Soll-Werten aus der Fahrablaufsteuerung im Nexonar-System ab."/2(y_soll)
  x_soll/1 -> "Zylindermotor-Ansteuerung Folgende Werte sind einstellbar: - Drehstaerke (in %) (-> ZM_pwm_out in \"Ausfuerung\") - Drehrichtung (rechts = 0, links = 1) (-> ZM_r_l_out in \"Init_und_Warten\") - Drehdauer (-> zwischen \"Ausfuehrung\" und \"Beendet\") - Ausfuehrungspunkt (in mm) [durch Wechsel der Soll-Position] (-> zwischen \"Init_und_Start\" und \"Ausfuehrung) Wichtig! Der Ausfuerungspunkt haengt von den EXAKTEN Soll-Werten aus der Fahrablaufsteuerung im Nexonar-System ab."/1(x_soll)

== system GesamtsystemAlt/Add-Ons-Eingang/Heckschalter-System ==
  Signaleingang fuer Heckschalter : c2833xlib/Digital Input  GPIO_Number=GPIO24~GPIO31  GPIO_Bit0=on  GPIO_Bit1=off  GPIO_Bit2=off  GPIO_Bit3=off  GPIO_Bit4=off  GPIO_Bit5=off  GPIO_Bit6=off  GPIO_Bit7=off  sampleTime=0.01  dataType=boolean  GPIO_Bit0_Qualification=Sync to SYSCLKOUT  GPIO_Bit1_Qualification=Sync to SYSCLKOUT  GPIO_Bit2_Qualification=Sync to SYSCLKOUT  GPIO_Bit3_Qualification=Sync to SYSCLKOUT  GPIO_Bit4_Qualification=Sync to SYSCLKOUT  GPIO_Bit5_Qualification=Sync to SYSCLKOUT  GPIO_Bit6_Qualification=Sync to SYSCLKOUT  GPIO_Bit7_Qualification=Sync to SYSCLKOUT  Qualification_Period=-1
      settings: SourceProductName=Embedded Coder Support Package for Texas Instruments C2000 Processors  SourceProductBaseCode=TIC2000
  Heckschalter : Outport
  wires:
  Signaleingang fuer Heckschalter/1 -> Heckschalter/1

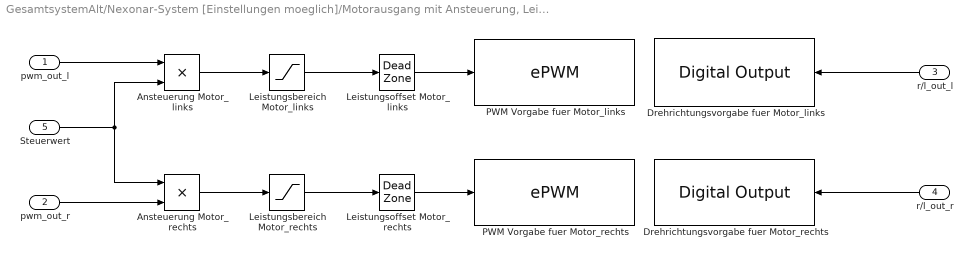
== system GesamtsystemAlt/Nexonar-System [Einstellungen moeglich]/Motorausgang mit Ansteuerung, Leistungsoffset und Leistungsregulierung ==
  pwm_out_l : Inport
  pwm_out_r : Inport  Port=2
  r/l_out_l : Inport  Port=3
  r/l_out_r : Inport  Port=4
  Steuerwert : Inport  Port=5
  Ansteuerung Motor_links : Product
  Ansteuerung Motor_rechts : Product
  Drehrichtungsvorgabe fuer Motor_links : c2833xlib/Digital Output  GPIO_Number=GPIO16~GPIO23  GPIO_Bit0=off  GPIO_BIT0_Toggle=off  GPIO_Bit1=off  GPIO_BIT1_Toggle=off  GPIO_Bit2=off  GPIO_BIT2_Toggle=off  GPIO_Bit3=off  GPIO_BIT3_Toggle=off  GPIO_Bit4=on  GPIO_BIT4_Toggle=off  GPIO_Bit5=off  GPIO_BIT5_Toggle=off  GPIO_Bit6=off  GPIO_BIT6_Toggle=off  GPIO_Bit7=off  GPIO_BIT7_Toggle=off
      settings: SourceProductName=Embedded Coder Support Package for Texas Instruments C2000 Processors  SourceProductBaseCode=TIC2000
  Drehrichtungsvorgabe fuer Motor_rechts : c2833xlib/Digital Output  GPIO_Number=GPIO16~GPIO23  GPIO_Bit0=off  GPIO_BIT0_Toggle=off  GPIO_Bit1=off  GPIO_BIT1_Toggle=off  GPIO_Bit2=off  GPIO_BIT2_Toggle=off  GPIO_Bit3=off  GPIO_BIT3_Toggle=off  GPIO_Bit4=off  GPIO_BIT4_Toggle=off  GPIO_Bit5=on  GPIO_BIT5_Toggle=off  GPIO_Bit6=off  GPIO_BIT6_Toggle=off  GPIO_Bit7=off  GPIO_BIT7_Toggle=off
      settings: SourceProductName=Embedded Coder Support Package for Texas Instruments C2000 Processors  SourceProductBaseCode=TIC2000
  Leistungsbereich Motor_links : Saturate  UpperLimit=80  LowerLimit=0
  Leistungsbereich Motor_rechts : Saturate  UpperLimit=80  LowerLimit=0
  Leistungsoffset Motor_links : DeadZone  LowerValue=0  UpperValue=0  SaturateOnIntegerOverflow=on
  Leistungsoffset Motor_rechts : DeadZone  LowerValue=0  UpperValue=3  SaturateOnIntegerOverflow=on
  "PWM Vorgabe fuer Motor_links " : c280xlib/ePWM  checkMode=off  useModule=ePWM1  periodUnits=Clock cycles  timerSource=Specify via dialog  timerPeriod_clk=64000  timerPeriod_sec=0.0001  tbshadow=Counter equals to zero  countingMode=Up  phaseActiveEnable=Disable  phaseDirection=Count down after sync  phaseActive=0  synchronizationEnable=off  synchronizationOption=Disable  clockPrescale=1  HSclockPrescale=1  ePWMxAStatus=off  CMPAUnits=Clock cycles  CMPASource=Specify via dialog  CMPAValue_per=50  CMPAValue_clk=32000  enCMPAshadow=Counter equals to zero  ePWMxAactionLogic1=Do nothing  ePWMxAactionLogic2=Clear  ePWMxAactionLogic3=Set  ePWMxAactionLogic4=Do nothing  ePWMxAactionLogic5=Do nothing  ePWMxAactionLogic6=Do nothing  ePWMxALoadMode=Load on counter equals to zero (CTR=Zero)  ePWMxACSFenable=off  ePWMxACSFvalue=Forcing disable  ePWMxASFreload=Zero  enHRPWM=off  HRPWM_LoadMode=Counter equals to zero (CTR=ZERO)  HRPWM_CTLMode=Phase control mode  HRPWM_EDGMode=Both edge  enSFO=on  ePWMxBStatus=on  CMPBUnits=Percentages  CMPBSource=Input port  CMPBValue_per=0  CMPBValue_clk=32000  enCMPBshadow=Counter equals to zero  ePWMxBactionLogic1=Do nothing  ePWMxBactionLogic2=Set  ePWMxBactionLogic3=Do nothing  ePWMxBactionLogic4=Do nothing  ePWMxBactionLogic5=Clear  ePWMxBactionLogic6=Do nothing  ePWMxBLoadMode=Load on counter equals to zero (CTR=Zero)  ePWMxBCSFenable=off  ePWMxBCSFvalue=Forcing disable  ePWMxBSFreload=Zero  enableDBePWMxA=off  enableDBePWMxB=off  DBpolarity=Active high (AH)  DBedgeDelay=Positive  DBSource_ePWMxA=ePWMxA  DBSource_ePWMxB=ePWMxA  DBperiodSource=Specify via dialog  REDperiod=0  FEDperiod=0  adcstartModuleA=off  adcrequestEventA=First event  adcstartEventA=Counter equals to zero (CTR=Zero)  adcstartModuleB=off  adcrequestEventB=First event  adcstartEventB=Counter equals to zero (CTR=Zero)  intEn=off  intPrd=First event  intSel=Counter equals to zero (CTR=Zero)  chopperEnable=off  chopperFrequency=1  chopperFirstwidth=1  chopperDuty=12.5%  tripZonesource=Specify via dialog  tzselOSHT1=off  tzselOSHT2=off  tzselOSHT3=off  tzselOSHT4=off  tzselOSHT5=off  tzselOSHT6=off  tzselCBC1=off  tzselCBC2=off  tzselCBC3=off  tzselCBC4=off  tzselCBC5=off  tzselCBC6=off  enTzOstIntr=off  enTzCbcIntr=off  ePWMxAforced=No action  ePWMxBforced=No action  timerPeriod=-1  ePWMxAValue=0  ePWMxBValue=0  tripZoneoption=One-shot trip (OSHT)
      settings: SourceProductName=Embedded Coder Support Package for Texas Instruments C2000 Processors  SourceProductBaseCode=TIC2000
  PWM Vorgabe fuer Motor_rechts : c280xlib/ePWM  checkMode=off  useModule=ePWM2  periodUnits=Clock cycles  timerSource=Specify via dialog  timerPeriod_clk=64000  timerPeriod_sec=0.0001  tbshadow=Counter equals to zero  countingMode=Up  phaseActiveEnable=Disable  phaseDirection=Count down after sync  phaseActive=0  synchronizationEnable=off  synchronizationOption=Disable  clockPrescale=1  HSclockPrescale=1  ePWMxAStatus=off  CMPAUnits=Clock cycles  CMPASource=Specify via dialog  CMPAValue_per=50  CMPAValue_clk=32000  enCMPAshadow=Counter equals to zero  ePWMxAactionLogic1=Do nothing  ePWMxAactionLogic2=Clear  ePWMxAactionLogic3=Set  ePWMxAactionLogic4=Do nothing  ePWMxAactionLogic5=Do nothing  ePWMxAactionLogic6=Do nothing  ePWMxALoadMode=Load on counter equals to zero (CTR=Zero)  ePWMxACSFenable=off  ePWMxACSFvalue=Forcing disable  ePWMxASFreload=Zero  enHRPWM=off  HRPWM_LoadMode=Counter equals to zero (CTR=ZERO)  HRPWM_CTLMode=Phase control mode  HRPWM_EDGMode=Both edge  enSFO=on  ePWMxBStatus=on  CMPBUnits=Percentages  CMPBSource=Input port  CMPBValue_per=0  CMPBValue_clk=32000  enCMPBshadow=Counter equals to zero  ePWMxBactionLogic1=Do nothing  ePWMxBactionLogic2=Set  ePWMxBactionLogic3=Do nothing  ePWMxBactionLogic4=Do nothing  ePWMxBactionLogic5=Clear  ePWMxBactionLogic6=Do nothing  ePWMxBLoadMode=Load on counter equals to zero (CTR=Zero)  ePWMxBCSFenable=off  ePWMxBCSFvalue=Forcing disable  ePWMxBSFreload=Zero  enableDBePWMxA=off  enableDBePWMxB=off  DBpolarity=Active high (AH)  DBedgeDelay=Positive  DBSource_ePWMxA=ePWMxA  DBSource_ePWMxB=ePWMxA  DBperiodSource=Specify via dialog  REDperiod=0  FEDperiod=0  adcstartModuleA=off  adcrequestEventA=First event  adcstartEventA=Counter equals to zero (CTR=Zero)  adcstartModuleB=off  adcrequestEventB=First event  adcstartEventB=Counter equals to zero (CTR=Zero)  intEn=off  intPrd=First event  intSel=Counter equals to zero (CTR=Zero)  chopperEnable=off  chopperFrequency=1  chopperFirstwidth=1  chopperDuty=12.5%  tripZonesource=Specify via dialog  tzselOSHT1=off  tzselOSHT2=off  tzselOSHT3=off  tzselOSHT4=off  tzselOSHT5=off  tzselOSHT6=off  tzselCBC1=off  tzselCBC2=off  tzselCBC3=off  tzselCBC4=off  tzselCBC5=off  tzselCBC6=off  enTzOstIntr=off  enTzCbcIntr=off  ePWMxAforced=No action  ePWMxBforced=No action  timerPeriod=-1  ePWMxAValue=0  ePWMxBValue=0  tripZoneoption=One-shot trip (OSHT)
      settings: SourceProductName=Embedded Coder Support Package for Texas Instruments C2000 Processors  SourceProductBaseCode=TIC2000
  wires:
  pwm_out_l/1 -> Ansteuerung Motor_links/1
  pwm_out_r/1 -> Ansteuerung Motor_rechts/2
  r/l_out_l/1 -> Drehrichtungsvorgabe fuer Motor_links/1
  r/l_out_r/1 -> Drehrichtungsvorgabe fuer Motor_rechts/1
  Leistungsoffset Motor_links/1 -> "PWM Vorgabe fuer Motor_links "/1
  Leistungsoffset Motor_rechts/1 -> PWM Vorgabe fuer Motor_rechts/1
  Steuerwert/1 -> Ansteuerung Motor_rechts/1, Ansteuerung Motor_links/2
  Ansteuerung Motor_rechts/1 -> Leistungsbereich Motor_rechts/1
  Leistungsbereich Motor_rechts/1 -> Leistungsoffset Motor_rechts/1
  Ansteuerung Motor_links/1 -> Leistungsbereich Motor_links/1
  Leistungsbereich Motor_links/1 -> Leistungsoffset Motor_links/1

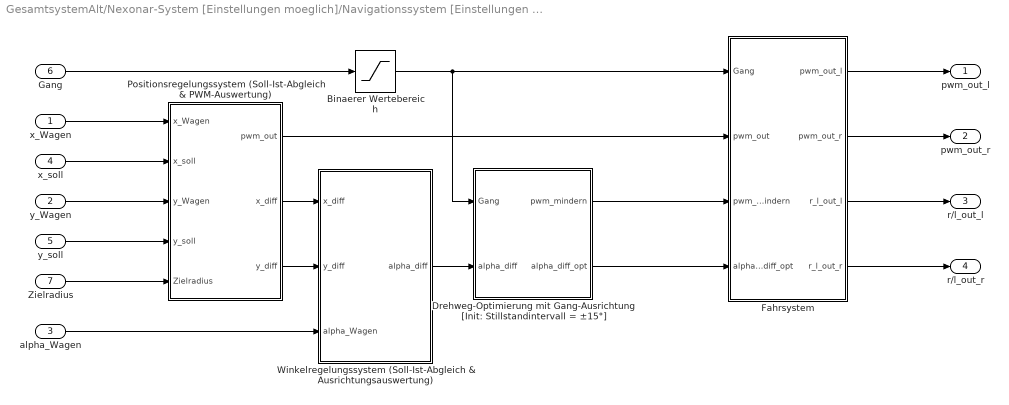
== system GesamtsystemAlt/Nexonar-System [Einstellungen moeglich]/Navigationssystem [Einstellungen moeglich] ==
  x_Wagen : Inport
  y_Wagen : Inport  Port=2
  alpha_Wagen : Inport  Port=3
  x_soll : Inport  Port=4
  y_soll : Inport  Port=5
  Gang : Inport  Port=6
  Zielradius : Inport  Port=7
  Binaerer Wertebereich : Saturate  UpperLimit=1  LowerLimit=0
  Drehweg-Optimierung mit Gang-Ausrichtung [Init: Stillstandintervall = ±15°] : Stateflow chart  TreatAsAtomicUnit=on
  Fahrsystem : Stateflow chart  TreatAsAtomicUnit=on
  Positionsregelungssystem (Soll-Ist-Abgleich & PWM-Auswertung) : Subsystem
  Winkelregelungssystem (Soll-Ist-Abgleich & Ausrichtungsauswertung) : Subsystem
  pwm_out_l : Outport
  pwm_out_r : Outport  Port=2
  r/l_out_l : Outport  Port=3
  r/l_out_r : Outport  Port=4
  wires:
  Positionsregelungssystem (Soll-Ist-Abgleich & PWM-Auswertung)/2(x_diff) -> Winkelregelungssystem (Soll-Ist-Abgleich & Ausrichtungsauswertung)/1(x_diff)
  y_soll/1 -> Positionsregelungssystem (Soll-Ist-Abgleich & PWM-Auswertung)/4(y_soll)
  y_Wagen/1 -> Positionsregelungssystem (Soll-Ist-Abgleich & PWM-Auswertung)/3(y_Wagen)
  Gang/1 -> Binaerer Wertebereich/1
  Positionsregelungssystem (Soll-Ist-Abgleich & PWM-Auswertung)/3(y_diff) -> Winkelregelungssystem (Soll-Ist-Abgleich & Ausrichtungsauswertung)/2(y_diff)
  x_Wagen/1 -> Positionsregelungssystem (Soll-Ist-Abgleich & PWM-Auswertung)/1(x_Wagen)
  x_soll/1 -> Positionsregelungssystem (Soll-Ist-Abgleich & PWM-Auswertung)/2(x_soll)
  alpha_Wagen/1 -> Winkelregelungssystem (Soll-Ist-Abgleich & Ausrichtungsauswertung)/3(alpha_Wagen)
  Fahrsystem/2(pwm_out_r) -> pwm_out_r/1
  Fahrsystem/4(r_l_out_r) -> r/l_out_r/1
  Fahrsystem/1(pwm_out_l) -> pwm_out_l/1
  Fahrsystem/3(r_l_out_l) -> r/l_out_l/1
  Winkelregelungssystem (Soll-Ist-Abgleich & Ausrichtungsauswertung)/1(alpha_diff) -> Drehweg-Optimierung mit Gang-Ausrichtung [Init: Stillstandintervall = ±15°]/2(alpha_diff)
  Drehweg-Optimierung mit Gang-Ausrichtung [Init: Stillstandintervall = ±15°]/2(alpha_diff_opt) -> Fahrsystem/4(alpha_diff_opt)
  Zielradius/1 -> Positionsregelungssystem (Soll-Ist-Abgleich & PWM-Auswertung)/5(Zielradius)
  Drehweg-Optimierung mit Gang-Ausrichtung [Init: Stillstandintervall = ±15°]/1(pwm_mindern) -> Fahrsystem/3(pwm_mindern)
  Positionsregelungssystem (Soll-Ist-Abgleich & PWM-Auswertung)/1(pwm_out) -> Fahrsystem/2(pwm_out)
  Binaerer Wertebereich/1 -> Fahrsystem/1(Gang), Drehweg-Optimierung mit Gang-Ausrichtung [Init: Stillstandintervall = ±15°]/1(Gang)

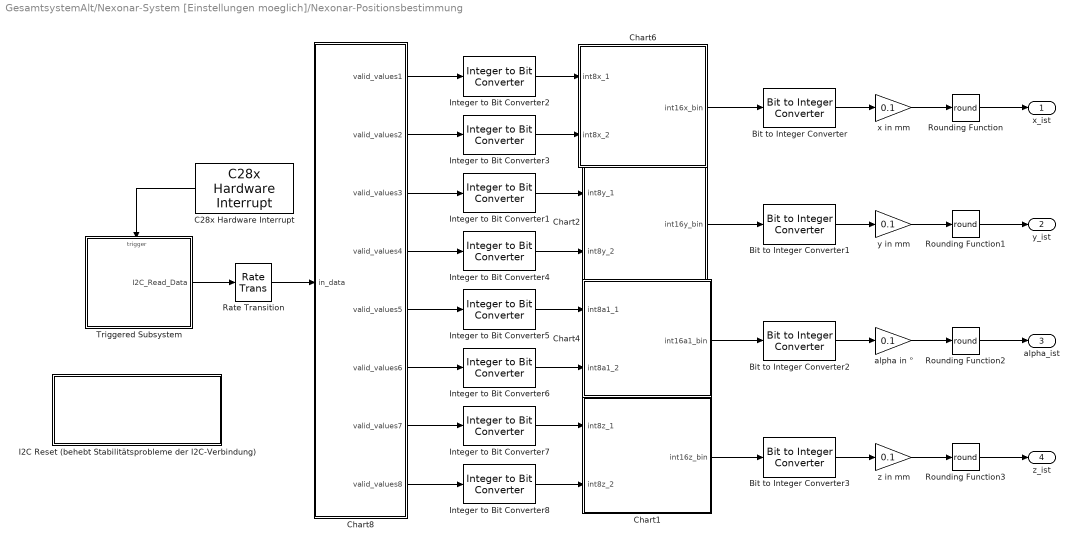
== system GesamtsystemAlt/Nexonar-System [Einstellungen moeglich]/Nexonar-Positionsbestimmung ==
  Bit to Integer Converter{,1..3} (4 alike) : commutil2/Bit to Integer Converter  nbits=16  bitOrder=MSB first  signedOutputValues=Signed  outDtype=Inherit via internal rule  outDtypeSigned=Inherit via internal rule
      settings: SourceProductName=Communications Toolbox
  C28x Hardware Interrupt : c2000lib/Scheduling/C28x Hardware Interrupt  irqnumbers=8  pienumbers=2  irqpriorities=30  irqpreempts=0  showinput=off  dspchiptype=C280X
      settings: SourceProductName=Embedded Coder Support Package for Texas Instruments C2000 Processors  SourceProductBaseCode=TIC2000
  Chart1 : Stateflow chart  TreatAsAtomicUnit=on
  Chart2 : Stateflow chart  TreatAsAtomicUnit=on
  Chart4 : Stateflow chart  TreatAsAtomicUnit=on
  Chart6 : Stateflow chart  TreatAsAtomicUnit=on
  Chart8 : Stateflow chart  TreatAsAtomicUnit=on
  I2C Reset (behebt Stabilitätsprobleme der I2C-Verbindung) : Subsystem
  Integer to Bit Converter{1..8} (8 alike) : commutil2/Integer to Bit Converter  nbits=8  signedInputValues=Unsigned  bitOrder=MSB first  outDtype=uint8
      settings: SourceProductName=Communications Toolbox
  Rate Transition : RateTransition  Deterministic=off  OutPortSampleTime=0.01
  Rounding Function{,1..3} (4 alike) : Rounding  Operator=round
  Triggered Subsystem : Subsystem  TreatAsAtomicUnit=on
  alpha in ° : Gain  Gain=0.1  OutDataTypeStr=double
  x in mm : Gain  Gain=0.1  OutDataTypeStr=double
  y in mm : Gain  Gain=0.1  OutDataTypeStr=double
  z in mm : Gain  Gain=0.1  OutDataTypeStr=double
  x_ist : Outport
  y_ist : Outport  Port=2
  alpha_ist : Outport  Port=3
  z_ist : Outport  Port=4
  wires:
  Integer to Bit Converter7/1 -> Chart1/1(int8z_1)
  Integer to Bit Converter8/1 -> Chart1/2(int8z_2)
  Chart8/7(valid_values7) -> Integer to Bit Converter7/1
  Chart8/8(valid_values8) -> Integer to Bit Converter8/1
  Triggered Subsystem/1(I2C_Read_Data) -> Rate Transition/1
  Chart1/1(int16z_bin) -> Bit to Integer Converter3/1
  Chart4/1(int16a1_bin) -> Bit to Integer Converter2/1
  Chart8/6(valid_values6) -> Integer to Bit Converter6/1
  Integer to Bit Converter6/1 -> Chart4/2(int8a1_2)
  Integer to Bit Converter5/1 -> Chart4/1(int8a1_1)
  Integer to Bit Converter4/1 -> Chart2/2(int8y_2)
  Integer to Bit Converter2/1 -> Chart6/1(int8x_1)
  Integer to Bit Converter1/1 -> Chart2/1(int8y_1)
  Chart6/1(int16x_bin) -> Bit to Integer Converter/1
  Integer to Bit Converter3/1 -> Chart6/2(int8x_2)
  Chart8/3(valid_values3) -> Integer to Bit Converter1/1
  Chart8/1(valid_values1) -> Integer to Bit Converter2/1
  Chart2/1(int16y_bin) -> Bit to Integer Converter1/1
  Chart8/4(valid_values4) -> Integer to Bit Converter4/1
  Chart8/2(valid_values2) -> Integer to Bit Converter3/1
  Chart8/5(valid_values5) -> Integer to Bit Converter5/1
  C28x Hardware Interrupt/1 -> Triggered Subsystem/Trigger
  Rate Transition/1 -> Chart8/1(in_data)
  x in mm/1 -> Rounding Function/1
  Bit to Integer Converter/1 -> x in mm/1
  Bit to Integer Converter1/1 -> y in mm/1
  y in mm/1 -> Rounding Function1/1
  Bit to Integer Converter3/1 -> z in mm/1
  z in mm/1 -> Rounding Function3/1
  Bit to Integer Converter2/1 -> alpha in °/1
  alpha in °/1 -> Rounding Function2/1
  Rounding Function/1 -> x_ist/1
  Rounding Function2/1 -> alpha_ist/1
  Rounding Function1/1 -> y_ist/1
  Rounding Function3/1 -> z_ist/1

== system GesamtsystemAlt/Subsystem/P-Regler mit Output2 ==
  Ist-Wert : Inport
  Soll-Wert : Inport  Port=2
  Drehrichtungsvorgabe für einen Motor : c2833xlib/Digital Output  GPIO_Number=GPIO16~GPIO23  GPIO_Bit0=off  GPIO_BIT0_Toggle=off  GPIO_Bit1=off  GPIO_BIT1_Toggle=off  GPIO_Bit2=off  GPIO_BIT2_Toggle=off  GPIO_Bit3=on  GPIO_BIT3_Toggle=off  GPIO_Bit4=off  GPIO_BIT4_Toggle=off  GPIO_Bit5=off  GPIO_BIT5_Toggle=off  GPIO_Bit6=off  GPIO_BIT6_Toggle=off  GPIO_Bit7=off  GPIO_BIT7_Toggle=off
      settings: SourceProductName=Embedded Coder Support Package for Texas Instruments C2000 Processors  SourceProductBaseCode=TIC2000
  "P-Regler mit Regelfehler Begrenzung Initial: k = 0.1, limiit = +/- 100 Sampletime 0.01" : Subsystem
  "PWM Vorgabe für einen Motor " : c280xlib/ePWM  checkMode=off  useModule=ePWM4  periodUnits=Clock cycles  timerSource=Specify via dialog  timerPeriod_clk=64000  timerPeriod_sec=0.0001  tbshadow=Counter equals to zero  countingMode=Up  phaseActiveEnable=Disable  phaseDirection=Count down after sync  phaseActive=0  synchronizationEnable=off  synchronizationOption=Disable  clockPrescale=1  HSclockPrescale=1  ePWMxAStatus=off  CMPAUnits=Clock cycles  CMPASource=Specify via dialog  CMPAValue_per=50  CMPAValue_clk=32000  enCMPAshadow=Counter equals to zero  ePWMxAactionLogic1=Do nothing  ePWMxAactionLogic2=Clear  ePWMxAactionLogic3=Set  ePWMxAactionLogic4=Do nothing  ePWMxAactionLogic5=Do nothing  ePWMxAactionLogic6=Do nothing  ePWMxALoadMode=Load on counter equals to zero (CTR=Zero)  ePWMxACSFenable=off  ePWMxACSFvalue=Forcing disable  ePWMxASFreload=Zero  enHRPWM=off  HRPWM_LoadMode=Counter equals to zero (CTR=ZERO)  HRPWM_CTLMode=Phase control mode  HRPWM_EDGMode=Both edge  enSFO=on  ePWMxBStatus=on  CMPBUnits=Percentages  CMPBSource=Input port  CMPBValue_per=0  CMPBValue_clk=32000  enCMPBshadow=Counter equals to zero  ePWMxBactionLogic1=Do nothing  ePWMxBactionLogic2=Set  ePWMxBactionLogic3=Do nothing  ePWMxBactionLogic4=Do nothing  ePWMxBactionLogic5=Clear  ePWMxBactionLogic6=Do nothing  ePWMxBLoadMode=Load on counter equals to zero (CTR=Zero)  ePWMxBCSFenable=off  ePWMxBCSFvalue=Forcing disable  ePWMxBSFreload=Zero  enableDBePWMxA=off  enableDBePWMxB=off  DBpolarity=Active high (AH)  DBedgeDelay=Positive  DBSource_ePWMxA=ePWMxA  DBSource_ePWMxB=ePWMxA  DBperiodSource=Specify via dialog  REDperiod=0  FEDperiod=0  adcstartModuleA=off  adcrequestEventA=First event  adcstartEventA=Counter equals to zero (CTR=Zero)  adcstartModuleB=off  adcrequestEventB=First event  adcstartEventB=Counter equals to zero (CTR=Zero)  intEn=off  intPrd=First event  intSel=Counter equals to zero (CTR=Zero)  chopperEnable=off  chopperFrequency=1  chopperFirstwidth=1  chopperDuty=12.5%  tripZonesource=Specify via dialog  tzselOSHT1=off  tzselOSHT2=off  tzselOSHT3=off  tzselOSHT4=off  tzselOSHT5=off  tzselOSHT6=off  tzselCBC1=off  tzselCBC2=off  tzselCBC3=off  tzselCBC4=off  tzselCBC5=off  tzselCBC6=off  enTzOstIntr=off  enTzCbcIntr=off  ePWMxAforced=No action  ePWMxBforced=No action  timerPeriod=-1  ePWMxAValue=0  ePWMxBValue=0  tripZoneoption=One-shot trip (OSHT)
      settings: SourceProductName=Embedded Coder Support Package for Texas Instruments C2000 Processors  SourceProductBaseCode=TIC2000
  wires:
  "P-Regler mit Regelfehler Begrenzung Initial: k = 0.1, limiit = +/- 100 Sampletime 0.01"/1(pwm_out) -> "PWM Vorgabe für einen Motor "/1
  "P-Regler mit Regelfehler Begrenzung Initial: k = 0.1, limiit = +/- 100 Sampletime 0.01"/2(r/l_out) -> Drehrichtungsvorgabe für einen Motor/1
  Soll-Wert/1 -> "P-Regler mit Regelfehler Begrenzung Initial: k = 0.1, limiit = +/- 100 Sampletime 0.01"/2(y_soll)
  Ist-Wert/1 -> "P-Regler mit Regelfehler Begrenzung Initial: k = 0.1, limiit = +/- 100 Sampletime 0.01"/1(y_ist)

== system GesamtsystemAlt/Subsystem/Subsystem2 ==
  In1 : Inport
  In2 : Inport  Port=2
  "Stopp " : Inport  Port=3
  Drehrichtungsvorgabe für einen Motor1 : c2833xlib/Digital Output  GPIO_Number=GPIO16~GPIO23  GPIO_Bit0=on  GPIO_BIT0_Toggle=off  GPIO_Bit1=off  GPIO_BIT1_Toggle=off  GPIO_Bit2=off  GPIO_BIT2_Toggle=off  GPIO_Bit3=off  GPIO_BIT3_Toggle=off  GPIO_Bit4=off  GPIO_BIT4_Toggle=off  GPIO_Bit5=off  GPIO_BIT5_Toggle=off  GPIO_Bit6=off  GPIO_BIT6_Toggle=off  GPIO_Bit7=off  GPIO_BIT7_Toggle=off
      settings: SourceProductName=Embedded Coder Support Package for Texas Instruments C2000 Processors  SourceProductBaseCode=TIC2000
  PWM Vorgabe für einen Motor 1 : c280xlib/ePWM  checkMode=off  useModule=ePWM6  periodUnits=Clock cycles  timerSource=Specify via dialog  timerPeriod_clk=64000  timerPeriod_sec=0.0001  tbshadow=Counter equals to zero  countingMode=Up  phaseActiveEnable=Disable  phaseDirection=Count down after sync  phaseActive=0  synchronizationEnable=off  synchronizationOption=Disable  clockPrescale=1  HSclockPrescale=1  ePWMxAStatus=off  CMPAUnits=Clock cycles  CMPASource=Specify via dialog  CMPAValue_per=50  CMPAValue_clk=32000  enCMPAshadow=Counter equals to zero  ePWMxAactionLogic1=Do nothing  ePWMxAactionLogic2=Clear  ePWMxAactionLogic3=Set  ePWMxAactionLogic4=Do nothing  ePWMxAactionLogic5=Do nothing  ePWMxAactionLogic6=Do nothing  ePWMxALoadMode=Load on counter equals to zero (CTR=Zero)  ePWMxACSFenable=off  ePWMxACSFvalue=Forcing disable  ePWMxASFreload=Zero  enHRPWM=off  HRPWM_LoadMode=Counter equals to zero (CTR=ZERO)  HRPWM_CTLMode=Phase control mode  HRPWM_EDGMode=Both edge  enSFO=on  ePWMxBStatus=on  CMPBUnits=Percentages  CMPBSource=Input port  CMPBValue_per=0  CMPBValue_clk=32000  enCMPBshadow=Counter equals to zero  ePWMxBactionLogic1=Do nothing  ePWMxBactionLogic2=Set  ePWMxBactionLogic3=Do nothing  ePWMxBactionLogic4=Do nothing  ePWMxBactionLogic5=Clear  ePWMxBactionLogic6=Do nothing  ePWMxBLoadMode=Load on counter equals to zero (CTR=Zero)  ePWMxBCSFenable=off  ePWMxBCSFvalue=Forcing disable  ePWMxBSFreload=Zero  enableDBePWMxA=off  enableDBePWMxB=off  DBpolarity=Active high (AH)  DBedgeDelay=Positive  DBSource_ePWMxA=ePWMxA  DBSource_ePWMxB=ePWMxA  DBperiodSource=Specify via dialog  REDperiod=0  FEDperiod=0  adcstartModuleA=off  adcrequestEventA=First event  adcstartEventA=Counter equals to zero (CTR=Zero)  adcstartModuleB=off  adcrequestEventB=First event  adcstartEventB=Counter equals to zero (CTR=Zero)  intEn=off  intPrd=First event  intSel=Counter equals to zero (CTR=Zero)  chopperEnable=off  chopperFrequency=1  chopperFirstwidth=1  chopperDuty=12.5%  tripZonesource=Specify via dialog  tzselOSHT1=off  tzselOSHT2=off  tzselOSHT3=off  tzselOSHT4=off  tzselOSHT5=off  tzselOSHT6=off  tzselCBC1=off  tzselCBC2=off  tzselCBC3=off  tzselCBC4=off  tzselCBC5=off  tzselCBC6=off  enTzOstIntr=off  enTzCbcIntr=off  ePWMxAforced=No action  ePWMxBforced=No action  timerPeriod=-1  ePWMxAValue=0  ePWMxBValue=0  tripZoneoption=One-shot trip (OSHT)
      settings: SourceProductName=Embedded Coder Support Package for Texas Instruments C2000 Processors  SourceProductBaseCode=TIC2000
  Product : Product
  wires:
  In2/1 -> Drehrichtungsvorgabe für einen Motor1/1
  Product/1 -> PWM Vorgabe für einen Motor 1/1
  In1/1 -> Product/2
  "Stopp "/1 -> Product/1
